simulink model "Simulacion_Repaso_Indivi_Masa_Restorte_Amort"  (R2016a)
settings: Solver=VariableStepAuto  StartTime=0.0  StopTime=70  RelTol=1e-3
undefined symbols (not defined in the file or in its folder): A, B, b1, b2, C, k1, k2, m1, m2
settings Model: Creator=Daniel  LastModifiedBy=Daniel

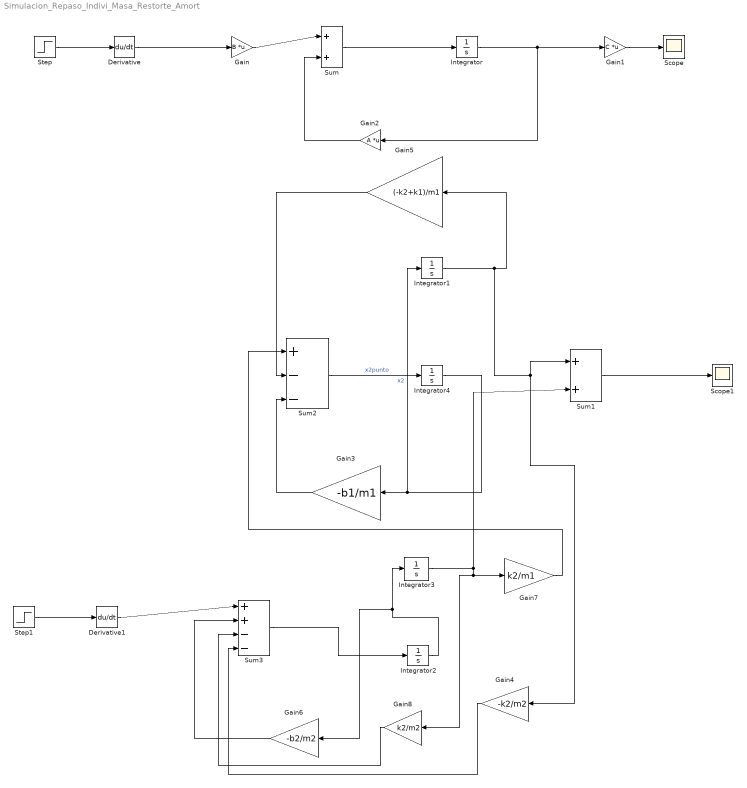
== system Simulacion_Repaso_Indivi_Masa_Restorte_Amort ==
  Derivative : Derivative
  Derivative1 : Derivative
  Gain : Gain  Gain=B  Multiplication=Matrix(K*u) (u vector)
  Gain1 : Gain  Gain=C  Multiplication=Matrix(K*u) (u vector)
  Gain2 : Gain  Gain=A  Multiplication=Matrix(K*u) (u vector)
  Gain3 : Gain  Gain=-b1/m1
  Gain4 : Gain  Gain=-k2/m2
  Gain5 : Gain  Gain=(-k2+k1)/m1
  Gain6 : Gain  Gain=-b2/m2
  Gain7 : Gain  Gain=k2/m1
  Gain8 : Gain  Gain=k2/m2
  Integrator{,1..4} (5 alike) : Integrator
  Scope : Scope
  Scope1 : Scope
  Step : Step  SampleTime=0
  Step1 : Step  SampleTime=0
  Sum : Sum  Inputs=|++
  Sum1 : Sum  Inputs=|++
  Sum2 : Sum  Inputs=|+--
  Sum3 : Sum  Inputs=|++--
  wires:
  Gain/1 -> Sum/1
  Sum/1 -> Integrator/1
  Integrator/1 -> Gain2/1, Gain1/1
  Gain2/1 -> Sum/2
  Step/1 -> Derivative/1
  Derivative/1 -> Gain/1
  Gain1/1 -> Scope/1
  Gain3/1 -> Sum2/3
  Sum2/1 -> Integrator4/1  "x2punto"
  Integrator4/1 -> Integrator1/1, Gain3/1  "x2"
  Gain5/1 -> Sum2/2
  Sum3/1 -> Integrator2/1
  Integrator2/1 -> Gain6/1, Integrator3/1
  Integrator3/1 -> Sum1/2, Gain7/1, Gain8/1
  Gain7/1 -> Sum2/1
  Integrator1/1 -> Gain4/1, Sum1/1, Gain5/1
  Gain4/1 -> Sum3/4
  Gain8/1 -> Sum3/3
  Gain6/1 -> Sum3/2
  Step1/1 -> Derivative1/1
  Derivative1/1 -> Sum3/1
  Sum1/1 -> Scope1/1
